simulink model "Microgrid_W"  (R2020a)
settings: Solver=ode15s  StartTime=0  StopTime=1440*1  MaxStep=1  RelTol=1e-3
libraries: simulink x4214, powerlib x685, simulink_extras x28, Microgrid_Library x18, powerlib_meascontrol x12
(part 27 of 48)

== system Microgrid_W/House 3 W3/Phone_Charger/D18 ==
  Add : Sum
  Clock : Clock
  Constant : Constant
  Constant1 : Constant  Value=0
  Gain : Gain  Gain=t
  Interval Test : simulink/Logic and Bit Operations/Interval Test  IntervalClosedRight=on  uplimit=Phone_C_3_Off_a+86400*4  IntervalClosedLeft=on  lowlimit=Phone_C_3_On_a+86400*4  OutDataTypeStr=boolean
  Interval Test1 : simulink/Logic and Bit Operations/Interval Test  IntervalClosedRight=on  uplimit=Phone_C_3_Off_b+86400*4  IntervalClosedLeft=on  lowlimit=Phone_C_3_On_b+86400*4  OutDataTypeStr=boolean
  Switch : Switch  Criteria=u2 > Threshold  Threshold=0.5
  Switch1 : Switch  Criteria=u2 > Threshold  Threshold=0.5
  Out1 : Outport  VectorParamsAs1DForOutWhenUnconnected=off
  wires:
  Gain/1 -> Interval Test/1, Interval Test1/1
  Switch1/1 -> Add/2
  Constant/1 -> Switch1/1, Switch/1
  Constant1/1 -> Switch1/3, Switch/3
  Add/1 -> Out1/1
  Interval Test1/1 -> Switch1/2
  Switch/1 -> Add/1
  Interval Test/1 -> Switch/2
  Clock/1 -> Gain/1

== system Microgrid_W/House 3 W3/Phone_Charger/D19 ==
  Add : Sum
  Clock : Clock
  Constant : Constant
  Constant1 : Constant  Value=0
  Gain : Gain  Gain=t
  Interval Test : simulink/Logic and Bit Operations/Interval Test  IntervalClosedRight=on  uplimit=Phone_C_3_Off_a+86400*5  IntervalClosedLeft=on  lowlimit=Phone_C_3_On_a+86400*5  OutDataTypeStr=boolean
  Interval Test1 : simulink/Logic and Bit Operations/Interval Test  IntervalClosedRight=on  uplimit=Phone_C_3_Off_b+86400*5  IntervalClosedLeft=on  lowlimit=Phone_C_3_On_b+86400*5  OutDataTypeStr=boolean
  Switch : Switch  Criteria=u2 > Threshold  Threshold=0.5
  Switch1 : Switch  Criteria=u2 > Threshold  Threshold=0.5
  Out1 : Outport  VectorParamsAs1DForOutWhenUnconnected=off
  wires:
  Interval Test/1 -> Switch/2
  Switch/1 -> Add/1
  Interval Test1/1 -> Switch1/2
  Add/1 -> Out1/1
  Constant1/1 -> Switch/3, Switch1/3
  Constant/1 -> Switch/1, Switch1/1
  Switch1/1 -> Add/2
  Gain/1 -> Interval Test1/1, Interval Test/1
  Clock/1 -> Gain/1

== system Microgrid_W/House 3 W3/Phone_Charger/D2 ==
  Add : Sum
  Clock : Clock
  Constant : Constant
  Constant1 : Constant  Value=0
  Gain : Gain  Gain=t
  Interval Test : simulink/Logic and Bit Operations/Interval Test  IntervalClosedRight=on  uplimit=Phone_C_1_Off_a+86400  IntervalClosedLeft=on  lowlimit=Phone_C_1_On_a+86400  OutDataTypeStr=boolean
  Interval Test1 : simulink/Logic and Bit Operations/Interval Test  IntervalClosedRight=on  uplimit=Phone_C_1_Off_b+86400  IntervalClosedLeft=on  lowlimit=Phone_C_1_On_b+86400  OutDataTypeStr=boolean
  Switch : Switch  Criteria=u2 > Threshold  Threshold=0.5
  Switch1 : Switch  Criteria=u2 > Threshold  Threshold=0.5
  Out1 : Outport  VectorParamsAs1DForOutWhenUnconnected=off
  wires:
  Interval Test/1 -> Switch/2
  Switch/1 -> Add/1
  Interval Test1/1 -> Switch1/2
  Add/1 -> Out1/1
  Constant1/1 -> Switch/3, Switch1/3
  Constant/1 -> Switch/1, Switch1/1
  Switch1/1 -> Add/2
  Gain/1 -> Interval Test1/1, Interval Test/1
  Clock/1 -> Gain/1

== system Microgrid_W/House 3 W3/Phone_Charger/D20 ==
  Add : Sum
  Clock : Clock
  Constant : Constant
  Constant1 : Constant  Value=0
  Gain : Gain  Gain=t
  Interval Test : simulink/Logic and Bit Operations/Interval Test  IntervalClosedRight=on  uplimit=Phone_C_3_Off_a  IntervalClosedLeft=on  lowlimit=Phone_C_3_On_a  OutDataTypeStr=boolean
  Interval Test1 : simulink/Logic and Bit Operations/Interval Test  IntervalClosedRight=on  uplimit=Phone_C_3_Off_b  IntervalClosedLeft=on  lowlimit=Phone_C_3_On_b  OutDataTypeStr=boolean
  Switch : Switch  Criteria=u2 > Threshold  Threshold=0.5
  Switch1 : Switch  Criteria=u2 > Threshold  Threshold=0.5
  Out1 : Outport  VectorParamsAs1DForOutWhenUnconnected=off
  wires:
  Gain/1 -> Interval Test/1, Interval Test1/1
  Switch1/1 -> Add/2
  Constant/1 -> Switch1/1, Switch/1
  Constant1/1 -> Switch1/3, Switch/3
  Add/1 -> Out1/1
  Interval Test1/1 -> Switch1/2
  Switch/1 -> Add/1
  Interval Test/1 -> Switch/2
  Clock/1 -> Gain/1

== system Microgrid_W/House 3 W3/Phone_Charger/D21 ==
  Add : Sum
  Clock : Clock
  Constant : Constant
  Constant1 : Constant  Value=0
  Gain : Gain  Gain=t
  Interval Test : simulink/Logic and Bit Operations/Interval Test  IntervalClosedRight=on  uplimit=Phone_C_3_Off_a+86400*6  IntervalClosedLeft=on  lowlimit=Phone_C_3_On_a+86400*6  OutDataTypeStr=boolean
  Interval Test1 : simulink/Logic and Bit Operations/Interval Test  IntervalClosedRight=on  uplimit=Phone_C_3_Off_b+86400*6  IntervalClosedLeft=on  lowlimit=Phone_C_3_On_b+86400*6  OutDataTypeStr=boolean
  Switch : Switch  Criteria=u2 > Threshold  Threshold=0.5
  Switch1 : Switch  Criteria=u2 > Threshold  Threshold=0.5
  Out1 : Outport  VectorParamsAs1DForOutWhenUnconnected=off
  wires:
  Gain/1 -> Interval Test/1, Interval Test1/1
  Switch1/1 -> Add/2
  Constant/1 -> Switch1/1, Switch/1
  Constant1/1 -> Switch1/3, Switch/3
  Add/1 -> Out1/1
  Interval Test1/1 -> Switch1/2
  Switch/1 -> Add/1
  Interval Test/1 -> Switch/2
  Clock/1 -> Gain/1

== system Microgrid_W/House 3 W3/Phone_Charger/D3 ==
  Add : Sum
  Clock : Clock
  Constant : Constant
  Constant1 : Constant  Value=0
  Gain : Gain  Gain=t
  Interval Test : simulink/Logic and Bit Operations/Interval Test  IntervalClosedRight=on  uplimit=Phone_C_1_Off_a+86400*2  IntervalClosedLeft=on  lowlimit=Phone_C_1_On_a+86400*2  OutDataTypeStr=boolean
  Interval Test1 : simulink/Logic and Bit Operations/Interval Test  IntervalClosedRight=on  uplimit=Phone_C_1_Off_b+86400*2  IntervalClosedLeft=on  lowlimit=Phone_C_1_On_b+86400*2  OutDataTypeStr=boolean
  Switch : Switch  Criteria=u2 > Threshold  Threshold=0.5
  Switch1 : Switch  Criteria=u2 > Threshold  Threshold=0.5
  Out1 : Outport  VectorParamsAs1DForOutWhenUnconnected=off
  wires:
  Gain/1 -> Interval Test/1, Interval Test1/1
  Switch1/1 -> Add/2
  Constant/1 -> Switch1/1, Switch/1
  Constant1/1 -> Switch1/3, Switch/3
  Add/1 -> Out1/1
  Interval Test1/1 -> Switch1/2
  Switch/1 -> Add/1
  Interval Test/1 -> Switch/2
  Clock/1 -> Gain/1

== system Microgrid_W/House 3 W3/Phone_Charger/D4 ==
  Add : Sum
  Clock : Clock
  Constant : Constant
  Constant1 : Constant  Value=0
  Gain : Gain  Gain=t
  Interval Test : simulink/Logic and Bit Operations/Interval Test  IntervalClosedRight=on  uplimit=Phone_C_1_Off_a+86400*3  IntervalClosedLeft=on  lowlimit=Phone_C_1_On_a+86400*3  OutDataTypeStr=boolean
  Interval Test1 : simulink/Logic and Bit Operations/Interval Test  IntervalClosedRight=on  uplimit=Phone_C_1_Off_b+86400*3  IntervalClosedLeft=on  lowlimit=Phone_C_1_On_b+86400*3  OutDataTypeStr=boolean
  Switch : Switch  Criteria=u2 > Threshold  Threshold=0.5
  Switch1 : Switch  Criteria=u2 > Threshold  Threshold=0.5
  Out1 : Outport  VectorParamsAs1DForOutWhenUnconnected=off
  wires:
  Interval Test/1 -> Switch/2
  Switch/1 -> Add/1
  Interval Test1/1 -> Switch1/2
  Add/1 -> Out1/1
  Constant1/1 -> Switch/3, Switch1/3
  Constant/1 -> Switch/1, Switch1/1
  Switch1/1 -> Add/2
  Gain/1 -> Interval Test1/1, Interval Test/1
  Clock/1 -> Gain/1

== system Microgrid_W/House 3 W3/Phone_Charger/D5 ==
  Add : Sum
  Clock : Clock
  Constant : Constant
  Constant1 : Constant  Value=0
  Gain : Gain  Gain=t
  Interval Test : simulink/Logic and Bit Operations/Interval Test  IntervalClosedRight=on  uplimit=Phone_C_1_Off_a+86400*4  IntervalClosedLeft=on  lowlimit=Phone_C_1_On_a+86400*4  OutDataTypeStr=boolean
  Interval Test1 : simulink/Logic and Bit Operations/Interval Test  IntervalClosedRight=on  uplimit=Phone_C_1_Off_b+86400*4  IntervalClosedLeft=on  lowlimit=Phone_C_1_On_b+86400*4  OutDataTypeStr=boolean
  Switch : Switch  Criteria=u2 > Threshold  Threshold=0.5
  Switch1 : Switch  Criteria=u2 > Threshold  Threshold=0.5
  Out1 : Outport  VectorParamsAs1DForOutWhenUnconnected=off
  wires:
  Gain/1 -> Interval Test/1, Interval Test1/1
  Switch1/1 -> Add/2
  Constant/1 -> Switch1/1, Switch/1
  Constant1/1 -> Switch1/3, Switch/3
  Add/1 -> Out1/1
  Interval Test1/1 -> Switch1/2
  Switch/1 -> Add/1
  Interval Test/1 -> Switch/2
  Clock/1 -> Gain/1

== system Microgrid_W/House 3 W3/Phone_Charger/D6 ==
  Add : Sum
  Clock : Clock
  Constant : Constant
  Constant1 : Constant  Value=0
  Gain : Gain  Gain=t
  Interval Test : simulink/Logic and Bit Operations/Interval Test  IntervalClosedRight=on  uplimit=Phone_C_1_Off_a+86400*5  IntervalClosedLeft=on  lowlimit=Phone_C_1_On_a+86400*5  OutDataTypeStr=boolean
  Interval Test1 : simulink/Logic and Bit Operations/Interval Test  IntervalClosedRight=on  uplimit=Phone_C_1_Off_b+86400*5  IntervalClosedLeft=on  lowlimit=Phone_C_1_On_b+86400*5  OutDataTypeStr=boolean
  Switch : Switch  Criteria=u2 > Threshold  Threshold=0.5
  Switch1 : Switch  Criteria=u2 > Threshold  Threshold=0.5
  Out1 : Outport  VectorParamsAs1DForOutWhenUnconnected=off
  wires:
  Interval Test/1 -> Switch/2
  Switch/1 -> Add/1
  Interval Test1/1 -> Switch1/2
  Add/1 -> Out1/1
  Constant1/1 -> Switch/3, Switch1/3
  Constant/1 -> Switch/1, Switch1/1
  Switch1/1 -> Add/2
  Gain/1 -> Interval Test1/1, Interval Test/1
  Clock/1 -> Gain/1

== system Microgrid_W/House 3 W3/Phone_Charger/D7 ==
  Add : Sum
  Clock : Clock
  Constant : Constant
  Constant1 : Constant  Value=0
  Gain : Gain  Gain=t
  Interval Test : simulink/Logic and Bit Operations/Interval Test  IntervalClosedRight=on  uplimit=Phone_C_1_Off_a+86400*6  IntervalClosedLeft=on  lowlimit=Phone_C_1_On_a+86400*6  OutDataTypeStr=boolean
  Interval Test1 : simulink/Logic and Bit Operations/Interval Test  IntervalClosedRight=on  uplimit=Phone_C_1_Off_b+86400*6  IntervalClosedLeft=on  lowlimit=Phone_C_1_On_b+86400*6  OutDataTypeStr=boolean
  Switch : Switch  Criteria=u2 > Threshold  Threshold=0.5
  Switch1 : Switch  Criteria=u2 > Threshold  Threshold=0.5
  Out1 : Outport  VectorParamsAs1DForOutWhenUnconnected=off
  wires:
  Gain/1 -> Interval Test/1, Interval Test1/1
  Switch1/1 -> Add/2
  Constant/1 -> Switch1/1, Switch/1
  Constant1/1 -> Switch1/3, Switch/3
  Add/1 -> Out1/1
  Interval Test1/1 -> Switch1/2
  Switch/1 -> Add/1
  Interval Test/1 -> Switch/2
  Clock/1 -> Gain/1

== system Microgrid_W/House 3 W3/Phone_Charger/D8 ==
  Add : Sum
  Clock : Clock
  Constant : Constant
  Constant1 : Constant  Value=0
  Gain : Gain  Gain=t
  Interval Test : simulink/Logic and Bit Operations/Interval Test  IntervalClosedRight=on  uplimit=Phone_C_2_Off_a  IntervalClosedLeft=on  lowlimit=Phone_C_2_On_a  OutDataTypeStr=boolean
  Interval Test1 : simulink/Logic and Bit Operations/Interval Test  IntervalClosedRight=on  uplimit=Phone_C_2_Off_b  IntervalClosedLeft=on  lowlimit=Phone_C_2_On_b  OutDataTypeStr=boolean
  Switch : Switch  Criteria=u2 > Threshold  Threshold=0.5
  Switch1 : Switch  Criteria=u2 > Threshold  Threshold=0.5
  Out1 : Outport  VectorParamsAs1DForOutWhenUnconnected=off
  wires:
  Interval Test/1 -> Switch/2
  Switch/1 -> Add/1
  Interval Test1/1 -> Switch1/2
  Add/1 -> Out1/1
  Constant1/1 -> Switch/3, Switch1/3
  Constant/1 -> Switch/1, Switch1/1
  Switch1/1 -> Add/2
  Gain/1 -> Interval Test1/1, Interval Test/1
  Clock/1 -> Gain/1

== system Microgrid_W/House 3 W3/Phone_Charger/D9 ==
  Add : Sum
  Clock : Clock
  Constant : Constant
  Constant1 : Constant  Value=0
  Gain : Gain  Gain=t
  Interval Test : simulink/Logic and Bit Operations/Interval Test  IntervalClosedRight=on  uplimit=Phone_C_2_Off_a+86400  IntervalClosedLeft=on  lowlimit=Phone_C_2_On_a+86400  OutDataTypeStr=boolean
  Interval Test1 : simulink/Logic and Bit Operations/Interval Test  IntervalClosedRight=on  uplimit=Phone_C_2_Off_b+86400  IntervalClosedLeft=on  lowlimit=Phone_C_2_On_b+86400  OutDataTypeStr=boolean
  Switch : Switch  Criteria=u2 > Threshold  Threshold=0.5
  Switch1 : Switch  Criteria=u2 > Threshold  Threshold=0.5
  Out1 : Outport  VectorParamsAs1DForOutWhenUnconnected=off
  wires:
  Gain/1 -> Interval Test/1, Interval Test1/1
  Switch1/1 -> Add/2
  Constant/1 -> Switch1/1, Switch/1
  Constant1/1 -> Switch1/3, Switch/3
  Add/1 -> Out1/1
  Interval Test1/1 -> Switch1/2
  Switch/1 -> Add/1
  Interval Test/1 -> Switch/2
  Clock/1 -> Gain/1

== system Microgrid_W/House 3 W3/Refrigerator/Subsystem ==
  In1 : Inport
  Add : Sum
  Cc : Constant  Value=2.7
  Constant : Constant  Value=150
  Divide{,1..3} (4 alike) : Product  Inputs=*/
  Gain : Gain  Gain=1/(60)
  Integrator : Integrator
  Off : Constant  Value=0
  Product{,1..3} (4 alike) : Product
  Rec : Constant  Value=0.35
  Rec1 : Constant
  Ri : Constant  Value=2
  Scope : Scope
  Subtract : Sum  Inputs=++-
  Switch : Switch  Criteria=u2 > Threshold  Threshold=0.5
  Switch1 : Switch  Criteria=u2 > Threshold  Threshold=0.5
  T_I : Constant  Value=T_Initial
  Ta : Constant  Value=20
  Te : Constant  Value=-10
  Thermostat : Subsystem
  Watts : Constant  Value=Fridge_W
  Out1 : Outport  VectorParamsAs1DForOutWhenUnconnected=off
  wires:
  Subtract/1 -> Gain/1
  Switch/1 -> Product2/2
  Switch1/1 -> Subtract/1
  In1/1 -> Switch1/2
  Product/1 -> Divide1/2
  Product1/1 -> Product2/1, Divide2/2
  Ta/1 -> Divide2/1
  Watts/1 -> Divide/1
  Cc/1 -> Product1/2, Product/1
  Divide1/1 -> Product3/2
  Divide2/1 -> Subtract/2
  Constant/1 -> Divide/2
  Divide3/1 -> Subtract/3
  Divide/1 -> Product3/1
  Product2/1 -> Divide3/2
  Te/1 -> Divide1/1
  Thermostat/1(Out1) -> Out1/1, Switch/2
  Ri/1 -> Product1/1
  Rec/1 -> Switch/3, Product/2
  Off/1 -> Switch1/3
  Product3/1 -> Switch1/1
  Rec1/1 -> Switch/1
  Gain/1 -> Integrator/1
  Integrator/1 -> Add/1
  Add/1 -> Divide3/1, Scope/1, Thermostat/1(In1)
  T_I/1 -> Add/2

== system Microgrid_W/House 3 W3/Shower/D1 ==
  Add : Sum  Inputs=+++
  Clock : Clock
  Constant : Constant
  Constant1 : Constant  Value=0
  Gain : Gain  Gain=t
  Interval Test : simulink/Logic and Bit Operations/Interval Test  IntervalClosedRight=on  uplimit=Shower_On_a+Shower_L_a  IntervalClosedLeft=on  lowlimit=Shower_On_a  OutDataTypeStr=boolean
  Interval Test1 : simulink/Logic and Bit Operations/Interval Test  IntervalClosedRight=on  uplimit=Shower_On_b+Shower_L_b  IntervalClosedLeft=on  lowlimit=Shower_On_b  OutDataTypeStr=boolean
  Interval Test2 : simulink/Logic and Bit Operations/Interval Test  IntervalClosedRight=on  uplimit=Shower_On_c+Shower_L_c  IntervalClosedLeft=on  lowlimit=Shower_On_c  OutDataTypeStr=boolean
  Switch : Switch  Criteria=u2 > Threshold  Threshold=0.5
  Switch1 : Switch  Criteria=u2 > Threshold  Threshold=0.5
  Switch2 : Switch  Criteria=u2 > Threshold  Threshold=0.5
  Out1 : Outport  VectorParamsAs1DForOutWhenUnconnected=off
  wires:
  Constant1/1 -> Switch2/3, Switch1/3, Switch/3
  Constant/1 -> Switch1/1, Switch2/1, Switch/1
  Gain/1 -> Interval Test2/1, Interval Test1/1, Interval Test/1
  Switch/1 -> Add/1
  Switch1/1 -> Add/2
  Switch2/1 -> Add/3
  Interval Test1/1 -> Switch1/2
  Interval Test/1 -> Switch/2
  Interval Test2/1 -> Switch2/2
  Add/1 -> Out1/1
  Clock/1 -> Gain/1

== system Microgrid_W/House 3 W3/Shower/D2 ==
  Add : Sum  Inputs=+++
  Clock : Clock
  Constant : Constant
  Constant1 : Constant  Value=0
  Gain : Gain  Gain=t
  Interval Test : simulink/Logic and Bit Operations/Interval Test  IntervalClosedRight=on  uplimit=Shower_On_a+(Shower_L_a+86400)  IntervalClosedLeft=on  lowlimit=Shower_On_a+86400  OutDataTypeStr=boolean
  Interval Test1 : simulink/Logic and Bit Operations/Interval Test  IntervalClosedRight=on  uplimit=Shower_On_b+(Shower_L_b+86400)  IntervalClosedLeft=on  lowlimit=Shower_On_b+86400  OutDataTypeStr=boolean
  Interval Test2 : simulink/Logic and Bit Operations/Interval Test  IntervalClosedRight=on  uplimit=Shower_On_c+(Shower_L_c+86400)  IntervalClosedLeft=on  lowlimit=Shower_On_c+86400  OutDataTypeStr=boolean
  Switch : Switch  Criteria=u2 > Threshold  Threshold=0.5
  Switch1 : Switch  Criteria=u2 > Threshold  Threshold=0.5
  Switch2 : Switch  Criteria=u2 > Threshold  Threshold=0.5
  Out1 : Outport  VectorParamsAs1DForOutWhenUnconnected=off
  wires:
  Add/1 -> Out1/1
  Interval Test2/1 -> Switch2/2
  Interval Test/1 -> Switch/2
  Interval Test1/1 -> Switch1/2
  Switch2/1 -> Add/3
  Switch1/1 -> Add/2
  Switch/1 -> Add/1
  Gain/1 -> Interval Test/1, Interval Test1/1, Interval Test2/1
  Constant/1 -> Switch/1, Switch2/1, Switch1/1
  Constant1/1 -> Switch/3, Switch1/3, Switch2/3
  Clock/1 -> Gain/1

== system Microgrid_W/House 3 W3/Shower/D3 ==
  Add : Sum  Inputs=+++
  Clock : Clock
  Constant : Constant
  Constant1 : Constant  Value=0
  Gain : Gain  Gain=t
  Interval Test : simulink/Logic and Bit Operations/Interval Test  IntervalClosedRight=on  uplimit=Shower_On_a+(Shower_L_a+86400*2)  IntervalClosedLeft=on  lowlimit=Shower_On_a+86400*2  OutDataTypeStr=boolean
  Interval Test1 : simulink/Logic and Bit Operations/Interval Test  IntervalClosedRight=on  uplimit=Shower_On_b+(Shower_L_b+86400*2)  IntervalClosedLeft=on  lowlimit=Shower_On_b+86400*2  OutDataTypeStr=boolean
  Interval Test2 : simulink/Logic and Bit Operations/Interval Test  IntervalClosedRight=on  uplimit=Shower_On_c+(Shower_L_c+86400*2)  IntervalClosedLeft=on  lowlimit=Shower_On_c+86400*2  OutDataTypeStr=boolean
  Switch : Switch  Criteria=u2 > Threshold  Threshold=0.5
  Switch1 : Switch  Criteria=u2 > Threshold  Threshold=0.5
  Switch2 : Switch  Criteria=u2 > Threshold  Threshold=0.5
  Out1 : Outport  VectorParamsAs1DForOutWhenUnconnected=off
  wires:
  Constant1/1 -> Switch2/3, Switch1/3, Switch/3
  Constant/1 -> Switch1/1, Switch2/1, Switch/1
  Gain/1 -> Interval Test2/1, Interval Test1/1, Interval Test/1
  Switch/1 -> Add/1
  Switch1/1 -> Add/2
  Switch2/1 -> Add/3
  Interval Test1/1 -> Switch1/2
  Interval Test/1 -> Switch/2
  Interval Test2/1 -> Switch2/2
  Add/1 -> Out1/1
  Clock/1 -> Gain/1

== system Microgrid_W/House 3 W3/Shower/D4 ==
  Add : Sum  Inputs=+++
  Clock : Clock
  Constant : Constant
  Constant1 : Constant  Value=0
  Gain : Gain  Gain=t
  Interval Test : simulink/Logic and Bit Operations/Interval Test  IntervalClosedRight=on  uplimit=Shower_On_a+Shower_L_a+86400*3  IntervalClosedLeft=on  lowlimit=Shower_On_a+86400*3  OutDataTypeStr=boolean
  Interval Test1 : simulink/Logic and Bit Operations/Interval Test  IntervalClosedRight=on  uplimit=Shower_On_b+Shower_L_b+86400*3  IntervalClosedLeft=on  lowlimit=Shower_On_b+86400*3  OutDataTypeStr=boolean
  Interval Test2 : simulink/Logic and Bit Operations/Interval Test  IntervalClosedRight=on  uplimit=Shower_On_c+Shower_L_c+86400*3  IntervalClosedLeft=on  lowlimit=Shower_On_c+86400*3  OutDataTypeStr=boolean
  Switch : Switch  Criteria=u2 > Threshold  Threshold=0.5
  Switch1 : Switch  Criteria=u2 > Threshold  Threshold=0.5
  Switch2 : Switch  Criteria=u2 > Threshold  Threshold=0.5
  Out1 : Outport  VectorParamsAs1DForOutWhenUnconnected=off
  wires:
  Add/1 -> Out1/1
  Interval Test2/1 -> Switch2/2
  Interval Test/1 -> Switch/2
  Interval Test1/1 -> Switch1/2
  Switch2/1 -> Add/3
  Switch1/1 -> Add/2
  Switch/1 -> Add/1
  Gain/1 -> Interval Test/1, Interval Test1/1, Interval Test2/1
  Constant/1 -> Switch/1, Switch2/1, Switch1/1
  Constant1/1 -> Switch/3, Switch1/3, Switch2/3
  Clock/1 -> Gain/1

== system Microgrid_W/House 3 W3/Shower/D5 ==
  Add : Sum  Inputs=+++
  Clock : Clock
  Constant : Constant
  Constant1 : Constant  Value=0
  Gain : Gain  Gain=t
  Interval Test : simulink/Logic and Bit Operations/Interval Test  IntervalClosedRight=on  uplimit=Shower_On_a+Shower_L_a+86400*4  IntervalClosedLeft=on  lowlimit=Shower_On_a+86400*4  OutDataTypeStr=boolean
  Interval Test1 : simulink/Logic and Bit Operations/Interval Test  IntervalClosedRight=on  uplimit=Shower_On_b+Shower_L_b+86400*4  IntervalClosedLeft=on  lowlimit=Shower_On_b+86400*4  OutDataTypeStr=boolean
  Interval Test2 : simulink/Logic and Bit Operations/Interval Test  IntervalClosedRight=on  uplimit=Shower_On_c+Shower_L_c+86400*4  IntervalClosedLeft=on  lowlimit=Shower_On_c+86400*4  OutDataTypeStr=boolean
  Switch : Switch  Criteria=u2 > Threshold  Threshold=0.5
  Switch1 : Switch  Criteria=u2 > Threshold  Threshold=0.5
  Switch2 : Switch  Criteria=u2 > Threshold  Threshold=0.5
  Out1 : Outport  VectorParamsAs1DForOutWhenUnconnected=off
  wires:
  Constant1/1 -> Switch2/3, Switch1/3, Switch/3
  Constant/1 -> Switch1/1, Switch2/1, Switch/1
  Gain/1 -> Interval Test2/1, Interval Test1/1, Interval Test/1
  Switch/1 -> Add/1
  Switch1/1 -> Add/2
  Switch2/1 -> Add/3
  Interval Test1/1 -> Switch1/2
  Interval Test/1 -> Switch/2
  Interval Test2/1 -> Switch2/2
  Add/1 -> Out1/1
  Clock/1 -> Gain/1

== system Microgrid_W/House 3 W3/Shower/D6 ==
  Add : Sum  Inputs=+++
  Clock : Clock
  Constant : Constant
  Constant1 : Constant  Value=0
  Gain : Gain  Gain=t
  Interval Test : simulink/Logic and Bit Operations/Interval Test  IntervalClosedRight=on  uplimit=Shower_On_a+Shower_L_a+86400*5  IntervalClosedLeft=on  lowlimit=Shower_On_a+86400*5  OutDataTypeStr=boolean
  Interval Test1 : simulink/Logic and Bit Operations/Interval Test  IntervalClosedRight=on  uplimit=Shower_On_b+Shower_L_b+86400*5  IntervalClosedLeft=on  lowlimit=Shower_On_b+86400*5  OutDataTypeStr=boolean
  Interval Test2 : simulink/Logic and Bit Operations/Interval Test  IntervalClosedRight=on  uplimit=Shower_On_c+Shower_L_c+86400*5  IntervalClosedLeft=on  lowlimit=Shower_On_c+86400*5  OutDataTypeStr=boolean
  Switch : Switch  Criteria=u2 > Threshold  Threshold=0.5
  Switch1 : Switch  Criteria=u2 > Threshold  Threshold=0.5
  Switch2 : Switch  Criteria=u2 > Threshold  Threshold=0.5
  Out1 : Outport  VectorParamsAs1DForOutWhenUnconnected=off
  wires:
  Add/1 -> Out1/1
  Interval Test2/1 -> Switch2/2
  Interval Test/1 -> Switch/2
  Interval Test1/1 -> Switch1/2
  Switch2/1 -> Add/3
  Switch1/1 -> Add/2
  Switch/1 -> Add/1
  Gain/1 -> Interval Test/1, Interval Test1/1, Interval Test2/1
  Constant/1 -> Switch/1, Switch2/1, Switch1/1
  Constant1/1 -> Switch/3, Switch1/3, Switch2/3
  Clock/1 -> Gain/1

== system Microgrid_W/House 3 W3/Shower/D7 ==
  Add : Sum  Inputs=+++
  Clock : Clock
  Constant : Constant
  Constant1 : Constant  Value=0
  Gain : Gain  Gain=t
  Interval Test : simulink/Logic and Bit Operations/Interval Test  IntervalClosedRight=on  uplimit=Shower_On_a+Shower_L_a+86400*6  IntervalClosedLeft=on  lowlimit=Shower_On_a+86400*6  OutDataTypeStr=boolean
  Interval Test1 : simulink/Logic and Bit Operations/Interval Test  IntervalClosedRight=on  uplimit=Shower_On_b+Shower_L_b+86400*6  IntervalClosedLeft=on  lowlimit=Shower_On_b+86400*6  OutDataTypeStr=boolean
  Interval Test2 : simulink/Logic and Bit Operations/Interval Test  IntervalClosedRight=on  uplimit=Shower_On_c+Shower_L_c+86400*6  IntervalClosedLeft=on  lowlimit=Shower_On_c+86400*6  OutDataTypeStr=boolean
  Switch : Switch  Criteria=u2 > Threshold  Threshold=0.5
  Switch1 : Switch  Criteria=u2 > Threshold  Threshold=0.5
  Switch2 : Switch  Criteria=u2 > Threshold  Threshold=0.5
  Out1 : Outport  VectorParamsAs1DForOutWhenUnconnected=off
  wires:
  Constant1/1 -> Switch2/3, Switch1/3, Switch/3
  Constant/1 -> Switch1/1, Switch2/1, Switch/1
  Gain/1 -> Interval Test2/1, Interval Test1/1, Interval Test/1
  Switch/1 -> Add/1
  Switch1/1 -> Add/2
  Switch2/1 -> Add/3
  Interval Test1/1 -> Switch1/2
  Interval Test/1 -> Switch/2
  Interval Test2/1 -> Switch2/2
  Add/1 -> Out1/1
  Clock/1 -> Gain/1

== system Microgrid_W/House 3 W3/Stereo/D1 ==
  Clock : Clock
  Constant : Constant
  Constant1 : Constant  Value=0
  Gain : Gain  Gain=t
  Interval Test : simulink/Logic and Bit Operations/Interval Test  IntervalClosedRight=on  uplimit=Stereo_Off_1  IntervalClosedLeft=on  lowlimit=Stereo_On_1  OutDataTypeStr=boolean
  Switch : Switch  Criteria=u2 > Threshold  Threshold=0.5
  Out1 : Outport  VectorParamsAs1DForOutWhenUnconnected=off
  wires:
  Interval Test/1 -> Switch/2
  Switch/1 -> Out1/1
  Constant1/1 -> Switch/3
  Constant/1 -> Switch/1
  Gain/1 -> Interval Test/1
  Clock/1 -> Gain/1

== system Microgrid_W/House 3 W3/Stereo/D2 ==
  Clock : Clock
  Constant : Constant
  Constant1 : Constant  Value=0
  Gain : Gain  Gain=t
  Interval Test : simulink/Logic and Bit Operations/Interval Test  IntervalClosedRight=on  uplimit=Stereo_Off_1+86400  IntervalClosedLeft=on  lowlimit=Stereo_On_1+86400  OutDataTypeStr=boolean
  Switch : Switch  Criteria=u2 > Threshold  Threshold=0.5
  Out1 : Outport  VectorParamsAs1DForOutWhenUnconnected=off
  wires:
  Gain/1 -> Interval Test/1
  Constant/1 -> Switch/1
  Constant1/1 -> Switch/3
  Switch/1 -> Out1/1
  Interval Test/1 -> Switch/2
  Clock/1 -> Gain/1

== system Microgrid_W/House 3 W3/Stereo/D3 ==
  Clock : Clock
  Constant : Constant
  Constant1 : Constant  Value=0
  Gain : Gain  Gain=t
  Interval Test : simulink/Logic and Bit Operations/Interval Test  IntervalClosedRight=on  uplimit=Stereo_Off_1+86400*2  IntervalClosedLeft=on  lowlimit=Stereo_On_1+86400*2  OutDataTypeStr=boolean
  Switch : Switch  Criteria=u2 > Threshold  Threshold=0.5
  Out1 : Outport  VectorParamsAs1DForOutWhenUnconnected=off
  wires:
  Interval Test/1 -> Switch/2
  Switch/1 -> Out1/1
  Constant1/1 -> Switch/3
  Constant/1 -> Switch/1
  Gain/1 -> Interval Test/1
  Clock/1 -> Gain/1

== system Microgrid_W/House 3 W3/Stereo/D4 ==
  Clock : Clock
  Constant : Constant
  Constant1 : Constant  Value=0
  Gain : Gain  Gain=t
  Interval Test : simulink/Logic and Bit Operations/Interval Test  IntervalClosedRight=on  uplimit=Stereo_Off_1+86400*3  IntervalClosedLeft=on  lowlimit=Stereo_On_1+86400*3  OutDataTypeStr=boolean
  Switch : Switch  Criteria=u2 > Threshold  Threshold=0.5
  Out1 : Outport  VectorParamsAs1DForOutWhenUnconnected=off
  wires:
  Gain/1 -> Interval Test/1
  Constant/1 -> Switch/1
  Constant1/1 -> Switch/3
  Switch/1 -> Out1/1
  Interval Test/1 -> Switch/2
  Clock/1 -> Gain/1

== system Microgrid_W/House 3 W3/Stereo/D5 ==
  Clock : Clock
  Constant : Constant
  Constant1 : Constant  Value=0
  Gain : Gain  Gain=t
  Interval Test : simulink/Logic and Bit Operations/Interval Test  IntervalClosedRight=on  uplimit=Stereo_Off_1+86400*4  IntervalClosedLeft=on  lowlimit=Stereo_On_1+86400*4  OutDataTypeStr=boolean
  Switch : Switch  Criteria=u2 > Threshold  Threshold=0.5
  Out1 : Outport  VectorParamsAs1DForOutWhenUnconnected=off
  wires:
  Interval Test/1 -> Switch/2
  Switch/1 -> Out1/1
  Constant1/1 -> Switch/3
  Constant/1 -> Switch/1
  Gain/1 -> Interval Test/1
  Clock/1 -> Gain/1

== system Microgrid_W/House 3 W3/Stereo/D6 ==
  Clock : Clock
  Constant : Constant
  Constant1 : Constant  Value=0
  Gain : Gain  Gain=t
  Interval Test : simulink/Logic and Bit Operations/Interval Test  IntervalClosedRight=on  uplimit=Stereo_Off_1+86400*5  IntervalClosedLeft=on  lowlimit=Stereo_On_1+86400*5  OutDataTypeStr=boolean
  Switch : Switch  Criteria=u2 > Threshold  Threshold=0.5
  Out1 : Outport  VectorParamsAs1DForOutWhenUnconnected=off
  wires:
  Gain/1 -> Interval Test/1
  Constant/1 -> Switch/1
  Constant1/1 -> Switch/3
  Switch/1 -> Out1/1
  Interval Test/1 -> Switch/2
  Clock/1 -> Gain/1

== system Microgrid_W/House 3 W3/Stereo/D7 ==
  Clock : Clock
  Constant : Constant
  Constant1 : Constant  Value=0
  Gain : Gain  Gain=t
  Interval Test : simulink/Logic and Bit Operations/Interval Test  IntervalClosedRight=on  uplimit=Stereo_Off_1+86400*6  IntervalClosedLeft=on  lowlimit=Stereo_On_1+86400*6  OutDataTypeStr=boolean
  Switch : Switch  Criteria=u2 > Threshold  Threshold=0.5
  Out1 : Outport  VectorParamsAs1DForOutWhenUnconnected=off
  wires:
  Interval Test/1 -> Switch/2
  Switch/1 -> Out1/1
  Constant1/1 -> Switch/3
  Constant/1 -> Switch/1
  Gain/1 -> Interval Test/1
  Clock/1 -> Gain/1

== system Microgrid_W/House 3 W3/Toaster/D1 ==
  Add : Sum
  Clock : Clock
  Compare To Zero : simulink/Logic and Bit Operations/Compare To Zero  relop=>  OutDataTypeStr=boolean
  Compare To Zero1 : simulink/Logic and Bit Operations/Compare To Zero  relop=>  OutDataTypeStr=boolean
  Constant : Constant
  Constant1 : Constant  Value=0
  Constant2 : Constant  Value=0
  Constant3 : Constant  Value=Toaster_On_1
  Constant4 : Constant
  Constant5 : Constant  Value=0
  Constant6 : Constant  Value=Toaster_On_2
  Gain : Gain  Gain=t
  Interval Test : simulink/Logic and Bit Operations/Interval Test  IntervalClosedRight=on  uplimit=Toaster_On_1+180  IntervalClosedLeft=on  lowlimit=Toaster_On_1  OutDataTypeStr=boolean
  Interval Test1 : simulink/Logic and Bit Operations/Interval Test  IntervalClosedRight=on  uplimit=Toaster_On_2+180  IntervalClosedLeft=on  lowlimit=Toaster_On_2  OutDataTypeStr=boolean
  Switch{,1..2,4} (4 alike) : Switch  Criteria=u2 > Threshold  Threshold=0.5
  Out1 : Outport  VectorParamsAs1DForOutWhenUnconnected=off
  wires:
  Interval Test/1 -> Switch/2
  Constant1/1 -> Switch2/3, Switch/3
  Gain/1 -> Interval Test/1, Interval Test1/1
  Constant3/1 -> Compare To Zero/1
  Constant/1 -> Switch1/1
  Constant2/1 -> Switch1/3
  Compare To Zero/1 -> Switch1/2
  Switch1/1 -> Switch/1
  Interval Test1/1 -> Switch2/2
  Constant6/1 -> Compare To Zero1/1
  Constant4/1 -> Switch4/1
  Constant5/1 -> Switch4/3
  Compare To Zero1/1 -> Switch4/2
  Switch4/1 -> Switch2/1
  Switch/1 -> Add/1
  Switch2/1 -> Add/2
  Add/1 -> Out1/1
  Clock/1 -> Gain/1

== system Microgrid_W/House 3 W3/Toaster/D2 ==
  Add : Sum
  Clock : Clock
  Compare To Zero : simulink/Logic and Bit Operations/Compare To Zero  relop=>  OutDataTypeStr=boolean
  Compare To Zero1 : simulink/Logic and Bit Operations/Compare To Zero  relop=>  OutDataTypeStr=boolean
  Constant : Constant
  Constant1 : Constant  Value=0
  Constant2 : Constant  Value=0
  Constant3 : Constant  Value=Toaster_On_1
  Constant4 : Constant
  Constant5 : Constant  Value=0
  Constant6 : Constant  Value=Toaster_On_2
  Gain : Gain  Gain=t
  Interval Test : simulink/Logic and Bit Operations/Interval Test  IntervalClosedRight=on  uplimit=Toaster_On_1+180+86400  IntervalClosedLeft=on  lowlimit=Toaster_On_1+86400  OutDataTypeStr=boolean
  Interval Test1 : simulink/Logic and Bit Operations/Interval Test  IntervalClosedRight=on  uplimit=Toaster_On_2+180+86400  IntervalClosedLeft=on  lowlimit=Toaster_On_2+86400  OutDataTypeStr=boolean
  Switch{,1..2,4} (4 alike) : Switch  Criteria=u2 > Threshold  Threshold=0.5
  Out1 : Outport  VectorParamsAs1DForOutWhenUnconnected=off
  wires:
  Add/1 -> Out1/1
  Switch2/1 -> Add/2
  Switch/1 -> Add/1
  Switch4/1 -> Switch2/1
  Compare To Zero1/1 -> Switch4/2
  Constant5/1 -> Switch4/3
  Constant4/1 -> Switch4/1
  Constant6/1 -> Compare To Zero1/1
  Interval Test1/1 -> Switch2/2
  Switch1/1 -> Switch/1
  Compare To Zero/1 -> Switch1/2
  Constant2/1 -> Switch1/3
  Constant/1 -> Switch1/1
  Constant3/1 -> Compare To Zero/1
  Gain/1 -> Interval Test1/1, Interval Test/1
  Constant1/1 -> Switch/3, Switch2/3
  Interval Test/1 -> Switch/2
  Clock/1 -> Gain/1

== system Microgrid_W/House 3 W3/Toaster/D3 ==
  Add : Sum
  Clock : Clock
  Compare To Zero : simulink/Logic and Bit Operations/Compare To Zero  relop=>  OutDataTypeStr=boolean
  Compare To Zero1 : simulink/Logic and Bit Operations/Compare To Zero  relop=>  OutDataTypeStr=boolean
  Constant : Constant
  Constant1 : Constant  Value=0
  Constant2 : Constant  Value=0
  Constant3 : Constant  Value=Toaster_On_1
  Constant4 : Constant
  Constant5 : Constant  Value=0
  Constant6 : Constant  Value=Toaster_On_2
  Gain : Gain  Gain=t
  Interval Test : simulink/Logic and Bit Operations/Interval Test  IntervalClosedRight=on  uplimit=Toaster_On_1+180+86400*2  IntervalClosedLeft=on  lowlimit=Toaster_On_1+86400*2  OutDataTypeStr=boolean
  Interval Test1 : simulink/Logic and Bit Operations/Interval Test  IntervalClosedRight=on  uplimit=Toaster_On_2+180+86400*2  IntervalClosedLeft=on  lowlimit=Toaster_On_2+86400*2  OutDataTypeStr=boolean
  Switch{,1..2,4} (4 alike) : Switch  Criteria=u2 > Threshold  Threshold=0.5
  Out1 : Outport  VectorParamsAs1DForOutWhenUnconnected=off
  wires:
  Interval Test/1 -> Switch/2
  Constant1/1 -> Switch2/3, Switch/3
  Gain/1 -> Interval Test/1, Interval Test1/1
  Constant3/1 -> Compare To Zero/1
  Constant/1 -> Switch1/1
  Constant2/1 -> Switch1/3
  Compare To Zero/1 -> Switch1/2
  Switch1/1 -> Switch/1
  Interval Test1/1 -> Switch2/2
  Constant6/1 -> Compare To Zero1/1
  Constant4/1 -> Switch4/1
  Constant5/1 -> Switch4/3
  Compare To Zero1/1 -> Switch4/2
  Switch4/1 -> Switch2/1
  Switch/1 -> Add/1
  Switch2/1 -> Add/2
  Add/1 -> Out1/1
  Clock/1 -> Gain/1

== system Microgrid_W/House 3 W3/Toaster/D4 ==
  Add : Sum
  Clock : Clock
  Compare To Zero : simulink/Logic and Bit Operations/Compare To Zero  relop=>  OutDataTypeStr=boolean
  Compare To Zero1 : simulink/Logic and Bit Operations/Compare To Zero  relop=>  OutDataTypeStr=boolean
  Constant : Constant
  Constant1 : Constant  Value=0
  Constant2 : Constant  Value=0
  Constant3 : Constant  Value=Toaster_On_1
  Constant4 : Constant
  Constant5 : Constant  Value=0
  Constant6 : Constant  Value=Toaster_On_2
  Gain : Gain  Gain=t
  Interval Test : simulink/Logic and Bit Operations/Interval Test  IntervalClosedRight=on  uplimit=Toaster_On_1+180+86400*3  IntervalClosedLeft=on  lowlimit=Toaster_On_1+86400*3  OutDataTypeStr=boolean
  Interval Test1 : simulink/Logic and Bit Operations/Interval Test  IntervalClosedRight=on  uplimit=Toaster_On_2+180+86400*3  IntervalClosedLeft=on  lowlimit=Toaster_On_2+86400*3  OutDataTypeStr=boolean
  Switch{,1..2,4} (4 alike) : Switch  Criteria=u2 > Threshold  Threshold=0.5
  Out1 : Outport  VectorParamsAs1DForOutWhenUnconnected=off
  wires:
  Add/1 -> Out1/1
  Switch2/1 -> Add/2
  Switch/1 -> Add/1
  Switch4/1 -> Switch2/1
  Compare To Zero1/1 -> Switch4/2
  Constant5/1 -> Switch4/3
  Constant4/1 -> Switch4/1
  Constant6/1 -> Compare To Zero1/1
  Interval Test1/1 -> Switch2/2
  Switch1/1 -> Switch/1
  Compare To Zero/1 -> Switch1/2
  Constant2/1 -> Switch1/3
  Constant/1 -> Switch1/1
  Constant3/1 -> Compare To Zero/1
  Gain/1 -> Interval Test1/1, Interval Test/1
  Constant1/1 -> Switch/3, Switch2/3
  Interval Test/1 -> Switch/2
  Clock/1 -> Gain/1

== system Microgrid_W/House 3 W3/Toaster/D5 ==
  Add : Sum
  Clock : Clock
  Compare To Zero : simulink/Logic and Bit Operations/Compare To Zero  relop=>  OutDataTypeStr=boolean
  Compare To Zero1 : simulink/Logic and Bit Operations/Compare To Zero  relop=>  OutDataTypeStr=boolean
  Constant : Constant
  Constant1 : Constant  Value=0
  Constant2 : Constant  Value=0
  Constant3 : Constant  Value=Toaster_On_1
  Constant4 : Constant
  Constant5 : Constant  Value=0
  Constant6 : Constant  Value=Toaster_On_2
  Gain : Gain  Gain=t
  Interval Test : simulink/Logic and Bit Operations/Interval Test  IntervalClosedRight=on  uplimit=Toaster_On_1+180+86400*4  IntervalClosedLeft=on  lowlimit=Toaster_On_1+86400*4  OutDataTypeStr=boolean
  Interval Test1 : simulink/Logic and Bit Operations/Interval Test  IntervalClosedRight=on  uplimit=Toaster_On_2+180+86400*4  IntervalClosedLeft=on  lowlimit=Toaster_On_2+86400*4  OutDataTypeStr=boolean
  Switch{,1..2,4} (4 alike) : Switch  Criteria=u2 > Threshold  Threshold=0.5
  Out1 : Outport  VectorParamsAs1DForOutWhenUnconnected=off
  wires:
  Interval Test/1 -> Switch/2
  Constant1/1 -> Switch2/3, Switch/3
  Gain/1 -> Interval Test/1, Interval Test1/1
  Constant3/1 -> Compare To Zero/1
  Constant/1 -> Switch1/1
  Constant2/1 -> Switch1/3
  Compare To Zero/1 -> Switch1/2
  Switch1/1 -> Switch/1
  Interval Test1/1 -> Switch2/2
  Constant6/1 -> Compare To Zero1/1
  Constant4/1 -> Switch4/1
  Constant5/1 -> Switch4/3
  Compare To Zero1/1 -> Switch4/2
  Switch4/1 -> Switch2/1
  Switch/1 -> Add/1
  Switch2/1 -> Add/2
  Add/1 -> Out1/1
  Clock/1 -> Gain/1

== system Microgrid_W/House 3 W3/Toaster/D6 ==
  Add : Sum
  Clock : Clock
  Compare To Zero : simulink/Logic and Bit Operations/Compare To Zero  relop=>  OutDataTypeStr=boolean
  Compare To Zero1 : simulink/Logic and Bit Operations/Compare To Zero  relop=>  OutDataTypeStr=boolean
  Constant : Constant
  Constant1 : Constant  Value=0
  Constant2 : Constant  Value=0
  Constant3 : Constant  Value=Toaster_On_1
  Constant4 : Constant
  Constant5 : Constant  Value=0
  Constant6 : Constant  Value=Toaster_On_2
  Gain : Gain  Gain=t
  Interval Test : simulink/Logic and Bit Operations/Interval Test  IntervalClosedRight=on  uplimit=Toaster_On_1+180+86400*5  IntervalClosedLeft=on  lowlimit=Toaster_On_1+86400*5  OutDataTypeStr=boolean
  Interval Test1 : simulink/Logic and Bit Operations/Interval Test  IntervalClosedRight=on  uplimit=Toaster_On_2+180+86400*5  IntervalClosedLeft=on  lowlimit=Toaster_On_2+86400*5  OutDataTypeStr=boolean
  Switch{,1..2,4} (4 alike) : Switch  Criteria=u2 > Threshold  Threshold=0.5
  Out1 : Outport  VectorParamsAs1DForOutWhenUnconnected=off
  wires:
  Add/1 -> Out1/1
  Switch2/1 -> Add/2
  Switch/1 -> Add/1
  Switch4/1 -> Switch2/1
  Compare To Zero1/1 -> Switch4/2
  Constant5/1 -> Switch4/3
  Constant4/1 -> Switch4/1
  Constant6/1 -> Compare To Zero1/1
  Interval Test1/1 -> Switch2/2
  Switch1/1 -> Switch/1
  Compare To Zero/1 -> Switch1/2
  Constant2/1 -> Switch1/3
  Constant/1 -> Switch1/1
  Constant3/1 -> Compare To Zero/1
  Gain/1 -> Interval Test1/1, Interval Test/1
  Constant1/1 -> Switch/3, Switch2/3
  Interval Test/1 -> Switch/2
  Clock/1 -> Gain/1

== system Microgrid_W/House 3 W3/Toaster/D7 ==
  Add : Sum
  Clock : Clock
  Compare To Zero : simulink/Logic and Bit Operations/Compare To Zero  relop=>  OutDataTypeStr=boolean
  Compare To Zero1 : simulink/Logic and Bit Operations/Compare To Zero  relop=>  OutDataTypeStr=boolean
  Constant : Constant
  Constant1 : Constant  Value=0
  Constant2 : Constant  Value=0
  Constant3 : Constant  Value=Toaster_On_1
  Constant4 : Constant
  Constant5 : Constant  Value=0
  Constant6 : Constant  Value=Toaster_On_2
  Gain : Gain  Gain=t
  Interval Test : simulink/Logic and Bit Operations/Interval Test  IntervalClosedRight=on  uplimit=Toaster_On_1+180+86400*6  IntervalClosedLeft=on  lowlimit=Toaster_On_1+86400*6  OutDataTypeStr=boolean
  Interval Test1 : simulink/Logic and Bit Operations/Interval Test  IntervalClosedRight=on  uplimit=Toaster_On_2+180+86400*6  IntervalClosedLeft=on  lowlimit=Toaster_On_2+86400*6  OutDataTypeStr=boolean
  Switch{,1..2,4} (4 alike) : Switch  Criteria=u2 > Threshold  Threshold=0.5
  Out1 : Outport  VectorParamsAs1DForOutWhenUnconnected=off
  wires:
  Interval Test/1 -> Switch/2
  Constant1/1 -> Switch2/3, Switch/3
  Gain/1 -> Interval Test/1, Interval Test1/1
  Constant3/1 -> Compare To Zero/1
  Constant/1 -> Switch1/1
  Constant2/1 -> Switch1/3
  Compare To Zero/1 -> Switch1/2
  Switch1/1 -> Switch/1
  Interval Test1/1 -> Switch2/2
  Constant6/1 -> Compare To Zero1/1
  Constant4/1 -> Switch4/1
  Constant5/1 -> Switch4/3
  Compare To Zero1/1 -> Switch4/2
  Switch4/1 -> Switch2/1
  Switch/1 -> Add/1
  Switch2/1 -> Add/2
  Add/1 -> Out1/1
  Clock/1 -> Gain/1

== system Microgrid_W/House 3 W3/Tv/D1 ==
  Add : Sum
  Clock : Clock
  Constant : Constant
  Constant1 : Constant  Value=0
  Gain : Gain  Gain=t
  Interval Test : simulink/Logic and Bit Operations/Interval Test  IntervalClosedRight=on  uplimit=TV_Off_1  IntervalClosedLeft=on  lowlimit=TV_On_1  OutDataTypeStr=boolean
  Interval Test1 : simulink/Logic and Bit Operations/Interval Test  IntervalClosedRight=on  uplimit=TV_Off_2  IntervalClosedLeft=on  lowlimit=TV_On_2  OutDataTypeStr=boolean
  Switch : Switch  Criteria=u2 > Threshold  Threshold=0.5
  Switch1 : Switch  Criteria=u2 > Threshold  Threshold=0.5
  Out1 : Outport  VectorParamsAs1DForOutWhenUnconnected=off
  wires:
  Gain/1 -> Interval Test/1, Interval Test1/1
  Switch1/1 -> Add/2
  Constant/1 -> Switch1/1, Switch/1
  Constant1/1 -> Switch1/3, Switch/3
  Add/1 -> Out1/1
  Interval Test1/1 -> Switch1/2
  Switch/1 -> Add/1
  Interval Test/1 -> Switch/2
  Clock/1 -> Gain/1

== system Microgrid_W/House 3 W3/Tv/D2 ==
  Add : Sum
  Clock : Clock
  Constant : Constant
  Constant1 : Constant  Value=0
  Gain : Gain  Gain=t
  Interval Test : simulink/Logic and Bit Operations/Interval Test  IntervalClosedRight=on  uplimit=TV_Off_1+86400  IntervalClosedLeft=on  lowlimit=TV_On_1+86400  OutDataTypeStr=boolean
  Interval Test1 : simulink/Logic and Bit Operations/Interval Test  IntervalClosedRight=on  uplimit=TV_Off_2+86400  IntervalClosedLeft=on  lowlimit=TV_On_2+86400  OutDataTypeStr=boolean
  Switch : Switch  Criteria=u2 > Threshold  Threshold=0.5
  Switch1 : Switch  Criteria=u2 > Threshold  Threshold=0.5
  Out1 : Outport  VectorParamsAs1DForOutWhenUnconnected=off
  wires:
  Interval Test/1 -> Switch/2
  Switch/1 -> Add/1
  Interval Test1/1 -> Switch1/2
  Add/1 -> Out1/1
  Constant1/1 -> Switch/3, Switch1/3
  Constant/1 -> Switch/1, Switch1/1
  Switch1/1 -> Add/2
  Gain/1 -> Interval Test1/1, Interval Test/1
  Clock/1 -> Gain/1

== system Microgrid_W/House 3 W3/Tv/D3 ==
  Add : Sum
  Clock : Clock
  Constant : Constant
  Constant1 : Constant  Value=0
  Gain : Gain  Gain=t
  Interval Test : simulink/Logic and Bit Operations/Interval Test  IntervalClosedRight=on  uplimit=TV_Off_1+86400*2  IntervalClosedLeft=on  lowlimit=TV_On_1+86400*2  OutDataTypeStr=boolean
  Interval Test1 : simulink/Logic and Bit Operations/Interval Test  IntervalClosedRight=on  uplimit=TV_Off_2+86400*2  IntervalClosedLeft=on  lowlimit=TV_On_2+86400*2  OutDataTypeStr=boolean
  Switch : Switch  Criteria=u2 > Threshold  Threshold=0.5
  Switch1 : Switch  Criteria=u2 > Threshold  Threshold=0.5
  Out1 : Outport  VectorParamsAs1DForOutWhenUnconnected=off
  wires:
  Gain/1 -> Interval Test/1, Interval Test1/1
  Switch1/1 -> Add/2
  Constant/1 -> Switch1/1, Switch/1
  Constant1/1 -> Switch1/3, Switch/3
  Add/1 -> Out1/1
  Interval Test1/1 -> Switch1/2
  Switch/1 -> Add/1
  Interval Test/1 -> Switch/2
  Clock/1 -> Gain/1

== system Microgrid_W/House 3 W3/Tv/D4 ==
  Add : Sum
  Clock : Clock
  Constant : Constant
  Constant1 : Constant  Value=0
  Gain : Gain  Gain=t
  Interval Test : simulink/Logic and Bit Operations/Interval Test  IntervalClosedRight=on  uplimit=TV_Off_1+86400*3  IntervalClosedLeft=on  lowlimit=TV_On_1+86400*3  OutDataTypeStr=boolean
  Interval Test1 : simulink/Logic and Bit Operations/Interval Test  IntervalClosedRight=on  uplimit=TV_Off_2+86400*3  IntervalClosedLeft=on  lowlimit=TV_On_2+86400*3  OutDataTypeStr=boolean
  Switch : Switch  Criteria=u2 > Threshold  Threshold=0.5
  Switch1 : Switch  Criteria=u2 > Threshold  Threshold=0.5
  Out1 : Outport  VectorParamsAs1DForOutWhenUnconnected=off
  wires:
  Interval Test/1 -> Switch/2
  Switch/1 -> Add/1
  Interval Test1/1 -> Switch1/2
  Add/1 -> Out1/1
  Constant1/1 -> Switch/3, Switch1/3
  Constant/1 -> Switch/1, Switch1/1
  Switch1/1 -> Add/2
  Gain/1 -> Interval Test1/1, Interval Test/1
  Clock/1 -> Gain/1

== system Microgrid_W/House 3 W3/Tv/D5 ==
  Add : Sum
  Clock : Clock
  Constant : Constant
  Constant1 : Constant  Value=0
  Gain : Gain  Gain=t
  Interval Test : simulink/Logic and Bit Operations/Interval Test  IntervalClosedRight=on  uplimit=TV_Off_1+86400*4  IntervalClosedLeft=on  lowlimit=TV_On_1+86400*4  OutDataTypeStr=boolean
  Interval Test1 : simulink/Logic and Bit Operations/Interval Test  IntervalClosedRight=on  uplimit=TV_Off_2+86400*4  IntervalClosedLeft=on  lowlimit=TV_On_2+86400*4  OutDataTypeStr=boolean
  Switch : Switch  Criteria=u2 > Threshold  Threshold=0.5
  Switch1 : Switch  Criteria=u2 > Threshold  Threshold=0.5
  Out1 : Outport  VectorParamsAs1DForOutWhenUnconnected=off
  wires:
  Gain/1 -> Interval Test/1, Interval Test1/1
  Switch1/1 -> Add/2
  Constant/1 -> Switch1/1, Switch/1
  Constant1/1 -> Switch1/3, Switch/3
  Add/1 -> Out1/1
  Interval Test1/1 -> Switch1/2
  Switch/1 -> Add/1
  Interval Test/1 -> Switch/2
  Clock/1 -> Gain/1

== system Microgrid_W/House 3 W3/Tv/D6 ==
  Add : Sum
  Clock : Clock
  Constant : Constant
  Constant1 : Constant  Value=0
  Gain : Gain  Gain=t
  Interval Test : simulink/Logic and Bit Operations/Interval Test  IntervalClosedRight=on  uplimit=TV_Off_1+86400*5  IntervalClosedLeft=on  lowlimit=TV_On_1+86400*5  OutDataTypeStr=boolean
  Interval Test1 : simulink/Logic and Bit Operations/Interval Test  IntervalClosedRight=on  uplimit=TV_Off_2+86400*5  IntervalClosedLeft=on  lowlimit=TV_On_2+86400*5  OutDataTypeStr=boolean
  Switch : Switch  Criteria=u2 > Threshold  Threshold=0.5
  Switch1 : Switch  Criteria=u2 > Threshold  Threshold=0.5
  Out1 : Outport  VectorParamsAs1DForOutWhenUnconnected=off
  wires:
  Interval Test/1 -> Switch/2
  Switch/1 -> Add/1
  Interval Test1/1 -> Switch1/2
  Add/1 -> Out1/1
  Constant1/1 -> Switch/3, Switch1/3
  Constant/1 -> Switch/1, Switch1/1
  Switch1/1 -> Add/2
  Gain/1 -> Interval Test1/1, Interval Test/1
  Clock/1 -> Gain/1

== system Microgrid_W/House 3 W3/Tv/D7 ==
  Add : Sum
  Clock : Clock
  Constant : Constant
  Constant1 : Constant  Value=0
  Gain : Gain  Gain=t
  Interval Test : simulink/Logic and Bit Operations/Interval Test  IntervalClosedRight=on  uplimit=TV_Off_1+86400*6  IntervalClosedLeft=on  lowlimit=TV_On_1+86400*6  OutDataTypeStr=boolean
  Interval Test1 : simulink/Logic and Bit Operations/Interval Test  IntervalClosedRight=on  uplimit=TV_Off_2+86400*6  IntervalClosedLeft=on  lowlimit=TV_On_2+86400*6  OutDataTypeStr=boolean
  Switch : Switch  Criteria=u2 > Threshold  Threshold=0.5
  Switch1 : Switch  Criteria=u2 > Threshold  Threshold=0.5
  Out1 : Outport  VectorParamsAs1DForOutWhenUnconnected=off
  wires:
  Gain/1 -> Interval Test/1, Interval Test1/1
  Switch1/1 -> Add/2
  Constant/1 -> Switch1/1, Switch/1
  Constant1/1 -> Switch1/3, Switch/3
  Add/1 -> Out1/1
  Interval Test1/1 -> Switch1/2
  Switch/1 -> Add/1
  Interval Test/1 -> Switch/2
  Clock/1 -> Gain/1

== system Microgrid_W/House 3 W3/Water tank/Thermostat ==
  In1 : Inport
  Compare To Constant : simulink/Logic and Bit Operations/Compare To Constant  relop=>=  const=T_High_WH  OutDataTypeStr=boolean
  Compare To Constant1 : simulink/Logic and Bit Operations/Compare To Constant  relop=<=  const=T_Low_WH  OutDataTypeStr=boolean
  Constant : Constant  Value=0
  Constant1 : Constant
  S-R Flip-Flop : simulink_extras/Flip Flops/S-R Flip-Flop  initial_condition=0
  Switch : Switch  Criteria=u2 > Threshold  Threshold=0.5
  Out1 : Outport  VectorParamsAs1DForOutWhenUnconnected=off
  wires:
  In1/1 -> Compare To Constant1/1, Compare To Constant/1
  Compare To Constant/1 -> S-R Flip-Flop/2
  Compare To Constant1/1 -> S-R Flip-Flop/1
  S-R Flip-Flop/1 -> Switch/2
  Switch/1 -> Out1/1
  Constant1/1 -> Switch/1
  Constant/1 -> Switch/3

== system Microgrid_W/House 4 W1/Heater/D1 ==
  Clock : Clock
  Constant : Constant
  Constant1 : Constant  Value=0
  Gain : Gain  Gain=t
  Interval Test : simulink/Logic and Bit Operations/Interval Test  IntervalClosedRight=on  uplimit=Heater_Off_1  IntervalClosedLeft=on  lowlimit=Heater_On_1  OutDataTypeStr=boolean
  Switch : Switch  Criteria=u2 > Threshold  Threshold=0.5
  Out1 : Outport  VectorParamsAs1DForOutWhenUnconnected=off
  wires:
  Interval Test/1 -> Switch/2
  Switch/1 -> Out1/1
  Constant1/1 -> Switch/3
  Constant/1 -> Switch/1
  Gain/1 -> Interval Test/1
  Clock/1 -> Gain/1

== system Microgrid_W/House 4 W1/Heater/D2 ==
  Clock : Clock
  Constant : Constant
  Constant1 : Constant  Value=0
  Gain : Gain  Gain=t
  Interval Test : simulink/Logic and Bit Operations/Interval Test  IntervalClosedRight=on  uplimit=Heater_Off_1+86400  IntervalClosedLeft=on  lowlimit=Heater_On_1+86400  OutDataTypeStr=boolean
  Switch : Switch  Criteria=u2 > Threshold  Threshold=0.5
  Out1 : Outport  VectorParamsAs1DForOutWhenUnconnected=off
  wires:
  Constant/1 -> Switch/1
  Constant1/1 -> Switch/3
  Switch/1 -> Out1/1
  Interval Test/1 -> Switch/2
  Gain/1 -> Interval Test/1
  Clock/1 -> Gain/1

== system Microgrid_W/House 4 W1/Heater/D3 ==
  Clock : Clock
  Constant : Constant
  Constant1 : Constant  Value=0
  Gain : Gain  Gain=t
  Interval Test : simulink/Logic and Bit Operations/Interval Test  IntervalClosedRight=on  uplimit=Heater_Off_1+86400*2  IntervalClosedLeft=on  lowlimit=Heater_On_1+86400*2  OutDataTypeStr=boolean
  Switch : Switch  Criteria=u2 > Threshold  Threshold=0.5
  Out1 : Outport  VectorParamsAs1DForOutWhenUnconnected=off
  wires:
  Interval Test/1 -> Switch/2
  Switch/1 -> Out1/1
  Constant1/1 -> Switch/3
  Constant/1 -> Switch/1
  Gain/1 -> Interval Test/1
  Clock/1 -> Gain/1

== system Microgrid_W/House 4 W1/Heater/D4 ==
  Clock : Clock
  Constant : Constant
  Constant1 : Constant  Value=0
  Gain : Gain  Gain=t
  Interval Test : simulink/Logic and Bit Operations/Interval Test  IntervalClosedRight=on  uplimit=Heater_Off_1+86400*3  IntervalClosedLeft=on  lowlimit=Heater_On_1+86400*3  OutDataTypeStr=boolean
  Switch : Switch  Criteria=u2 > Threshold  Threshold=0.5
  Out1 : Outport  VectorParamsAs1DForOutWhenUnconnected=off
  wires:
  Constant/1 -> Switch/1
  Constant1/1 -> Switch/3
  Switch/1 -> Out1/1
  Interval Test/1 -> Switch/2
  Gain/1 -> Interval Test/1
  Clock/1 -> Gain/1

== system Microgrid_W/House 4 W1/Heater/D5 ==
  Clock : Clock
  Constant : Constant
  Constant1 : Constant  Value=0
  Gain : Gain  Gain=t
  Interval Test : simulink/Logic and Bit Operations/Interval Test  IntervalClosedRight=on  uplimit=Heater_Off_1+86400*4  IntervalClosedLeft=on  lowlimit=Heater_On_1+86400*4  OutDataTypeStr=boolean
  Switch : Switch  Criteria=u2 > Threshold  Threshold=0.5
  Out1 : Outport  VectorParamsAs1DForOutWhenUnconnected=off
  wires:
  Interval Test/1 -> Switch/2
  Switch/1 -> Out1/1
  Constant1/1 -> Switch/3
  Constant/1 -> Switch/1
  Gain/1 -> Interval Test/1
  Clock/1 -> Gain/1
